simulink model "BackgroundEst"  (Simulink 10.0)
settings: Solver=ode45  StartTime=0.0  StopTime=inf  RelTol=1e-3  EnableMultiTasking=on
undefined symbols (not defined in the file): High
libraries: vipsnks x3, simulink x3, dspsrcs4 x1, dspswit3 x1, dspsigops x1, vipconversions x1
settings Model: Creator=ahwang  LastModifiedBy=bhisma
settings SolverCC: ZeroCrossAlgorithm=Non-adaptive
settings DataIOCC: LimitDataPoints=on  SignalLoggingSaveFormat=ModelDataLogs
settings OptimizationCC: ExpressionDepthLimit=2147483647  InitFltsAndDblsToZero=on
settings DebuggingCC: SolverPrmCheckMsg=warning  FcnCallInpInsideContextMsg=warning  StateNameClashWarn=warning
settings SFSimCC: SimUseLocalCustomCode=on  SimParseCustomCode=off  CustomCodeUndefinedFunction=FilterOut
settings RTWCC: RTWUseLocalCustomCode=on

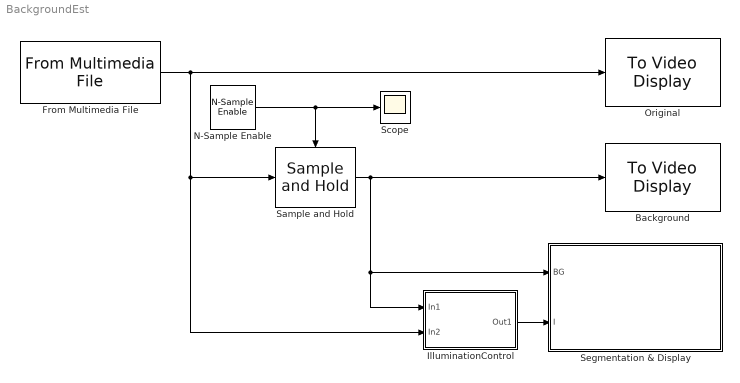
== system BackgroundEst ==
  Background : vipsnks/To Video Display  inputType=Obsolete  imagePorts=One multidimensional signal  OutputDevice=On-screen video monitor  fullScreen=off  videoWindowX=292  videoWindowY=180  saveWindowSize=off  videoWindowWidth=44  videoWindowHeight=41  dataOrg=Column-major
      settings: SourceProductName=Computer Vision Toolbox  SourceProductBaseCode=VP
  From Multimedia File : dspsrcs4/From Multimedia File  inputFilename=vipmen.avi  loop=on  numPlays=inf  outputStreams=Video only  videoDataType=double  audioDataType=int16  inheritSampleTime=on  userDefinedSampleTime=1/30  noAudioOutput=off  isIntensityVideo=on  colorVideoFormat=One multidimensional signal  outputEOF=off  dataOrg=Column-major
      settings: SourceProductName=DSP System Toolbox  SourceProductBaseCode=DS
  IlluminationControl : Subsystem
  N-Sample Enable : dspswit3/N-Sample Enable  N=1  ActiveLevel=High (1)  reset=off  TriggerType=Rising edge  Ts=-1  DataType=Logical
      settings: SourceProductName=DSP System Toolbox  SourceProductBaseCode=DS
  Original : vipsnks/To Video Display  inputType=Obsolete  imagePorts=One multidimensional signal  OutputDevice=On-screen video monitor  fullScreen=off  videoWindowX=292  videoWindowY=32  saveWindowSize=off  videoWindowWidth=44  videoWindowHeight=41  dataOrg=Column-major
      settings: SourceProductName=Computer Vision Toolbox  SourceProductBaseCode=VP
  Sample and Hold : dspsigops/Sample and Hold  SystemSampleTime=-1  trig=Rising edge  initCond=0  latchinput=off
  Scope : Scope
  Segmentation & Display : Subsystem
  wires:
  From Multimedia File/1 -> Original/1, Sample and Hold/1, IlluminationControl/2(In2)
  Sample and Hold/1 -> Background/1, Segmentation & Display/1(BG), IlluminationControl/1(In1)
  N-Sample Enable/1 -> Sample and Hold/Trigger, Scope/1
  IlluminationControl/1(Out1) -> Segmentation & Display/2(I)

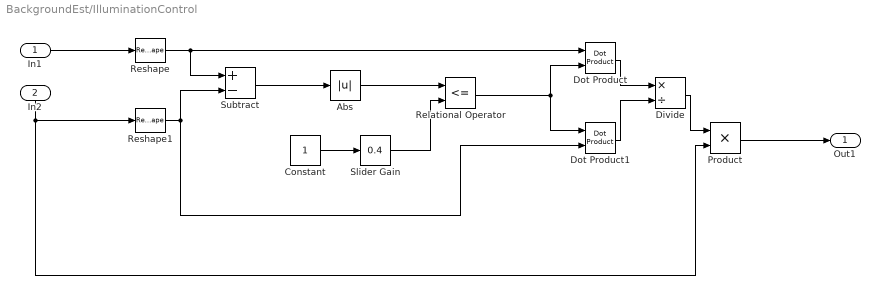
== system BackgroundEst/IlluminationControl ==
  In1 : Inport
  In2 : Inport  Port=2
  Abs : Abs
  Constant : Constant
  Divide : Product  Inputs=*/
  Dot Product : simulink/Math Operations/Dot Product  OutDataType=sfix(16)  OutScaling=2^-10  DoSatur=off
      settings: SourceProductName=Simulink  SourceProductBaseCode=SL
  Dot Product1 : simulink/Math Operations/Dot Product  OutDataType=sfix(16)  OutScaling=2^-10  DoSatur=off
      settings: SourceProductName=Simulink  SourceProductBaseCode=SL
  Product : Product  RndMeth=Zero
  Relational Operator : RelationalOperator  Operator=<=  OutDataTypeStr=boolean  RndMeth=Nearest
  Reshape : Reshape
  Reshape1 : Reshape
  Slider Gain : simulink/Math Operations/Slider Gain  SystemSampleTime=-1  low=0  gain=0.4  high=1
  Subtract : Sum  Inputs=+-
  Out1 : Outport
  wires:
  Subtract/1 -> Abs/1
  Reshape1/1 -> Subtract/2, Dot Product1/2
  Abs/1 -> Relational Operator/1
  Slider Gain/1 -> Relational Operator/2
  Constant/1 -> Slider Gain/1
  Relational Operator/1 -> Dot Product/2, Dot Product1/1
  Dot Product/1 -> Divide/1
  Dot Product1/1 -> Divide/2
  Divide/1 -> Product/1
  In1/1 -> Reshape/1
  Product/1 -> Out1/1
  Reshape/1 -> Subtract/1, Dot Product/1
  In2/1 -> Reshape1/1, Product/2

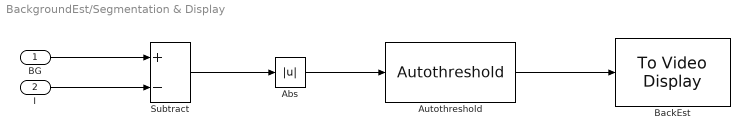
== system BackgroundEst/Segmentation & Display ==
  BG : Inport
  I : Inport  Port=2
  Abs : Abs
  Autothreshold : vipconversions/Autothreshold  operator=>  threshOut=off  effMetricOut=off  userDefinedRange=off  umin=0  umax=255  outOfRngOpt=Warn and saturate  scaleThreshold=off  scaleFactor=1  P1Mode=Specify word length  P1WordLength=32  P1FracLength=30  P2Mode=Specify word length  P2WordLength=32  P2FracLength=22  P3Mode=Specify word length  P3WordLength=32  P3FracLength=14  P4Mode=Binary point scaling  P4WordLength=32  P4FracLength=15  Q1Mode=Specify word length  Q1WordLength=32  Q1FracLength=16  EMMode=Specify word length  EMWordLength=16  EMFracLength=14  roundingMode=Floor  overflowMode=off
      settings: SourceProductName=Computer Vision Toolbox  SourceProductBaseCode=VP
  BackEst : vipsnks/To Video Display  inputType=Obsolete  imagePorts=One multidimensional signal  OutputDevice=On-screen video monitor  fullScreen=off  videoWindowX=290  videoWindowY=327  saveWindowSize=off  videoWindowWidth=44  videoWindowHeight=41  dataOrg=Column-major
      settings: SourceProductName=Computer Vision Toolbox  SourceProductBaseCode=VP
  Subtract : Sum  Inputs=+-
  wires:
  Subtract/1 -> Abs/1
  Autothreshold/1 -> BackEst/1
  BG/1 -> Subtract/1
  I/1 -> Subtract/2
  Abs/1 -> Autothreshold/1
